simulink model "Lab1_2_Integration_RLC"  (R2024b)
settings: Solver=FixedStepAuto  StartTime=0.0  StopTime=10.0  FixedStep=1e-3  RelTol=1e-3
undefined symbols (not defined in the file or in its folder): DiscIntNeverNeededParam
libraries: simulink x1
settings Model: Creator=Ahmad  LastModifiedBy=Ahmad

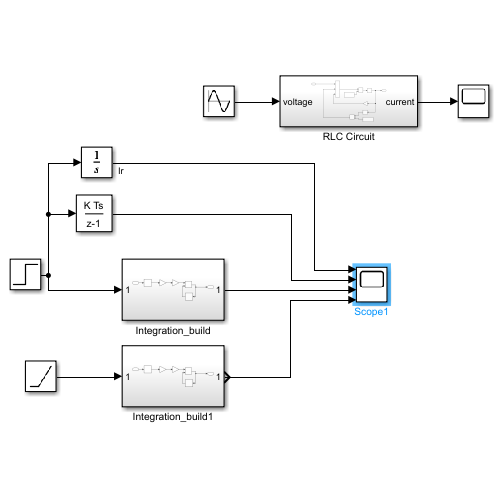
[thumbnail: Simulink's stored preview of the top-level diagram]
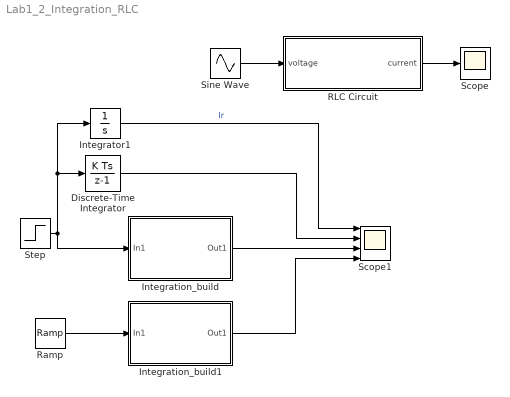
== system Lab1_2_Integration_RLC ==
  Discrete-Time Integrator : DiscreteIntegrator  SampleTime=-1  ICPrevOutput=DiscIntNeverNeededParam  ICPrevScaledInput=DiscIntNeverNeededParam
  Integration_build : Subsystem
  Integration_build1 : Subsystem
  Integrator1 : Integrator
  RLC Circuit : Subsystem
  Ramp : simulink/Sources/Ramp  slope=1  start=0  InitialOutput=0
  Scope : Scope
  Scope1 : Scope  NumInputPorts=4
  Sine Wave : Sin  SampleTime=0
  Step : Step  SampleTime=0
  wires:
  RLC Circuit/1(current) -> Scope/1
  Sine Wave/1 -> RLC Circuit/1(voltage)
  Step/1 -> Integration_build/1(In1), Discrete-Time Integrator/1, Integrator1/1
  Discrete-Time Integrator/1 -> Scope1/2
  Integrator1/1 -> Scope1/1  "Ir"
  Integration_build/1(Out1) -> Scope1/3
  Ramp/1 -> Integration_build1/1(In1)
  Integration_build1/1(Out1) -> Scope1/4

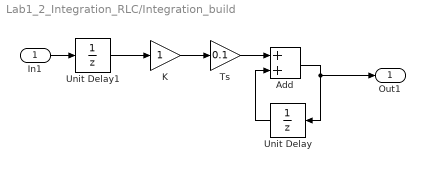
== system Lab1_2_Integration_RLC/Integration_build ==
  In1 : Inport
  Add : Sum
  K : Gain
  Ts : Gain  Gain=0.1
  Unit Delay : UnitDelay  SampleTime=-1  HasFrameUpgradeWarning=on
  Unit Delay1 : UnitDelay  SampleTime=-1  HasFrameUpgradeWarning=on
  Out1 : Outport
  wires:
  Ts/1 -> Add/1
  Unit Delay/1 -> Add/2
  In1/1 -> Unit Delay1/1
  K/1 -> Ts/1
  Add/1 -> Out1/1, Unit Delay/1
  Unit Delay1/1 -> K/1

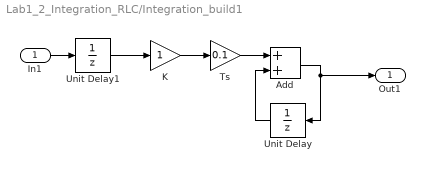
== system Lab1_2_Integration_RLC/Integration_build1 ==
  In1 : Inport
  Add : Sum
  K : Gain
  Ts : Gain  Gain=0.1
  Unit Delay : UnitDelay  SampleTime=-1  HasFrameUpgradeWarning=on
  Unit Delay1 : UnitDelay  SampleTime=-1  HasFrameUpgradeWarning=on
  Out1 : Outport
  wires:
  Ts/1 -> Add/1
  Unit Delay/1 -> Add/2
  In1/1 -> Unit Delay1/1
  K/1 -> Ts/1
  Add/1 -> Out1/1, Unit Delay/1
  Unit Delay1/1 -> K/1

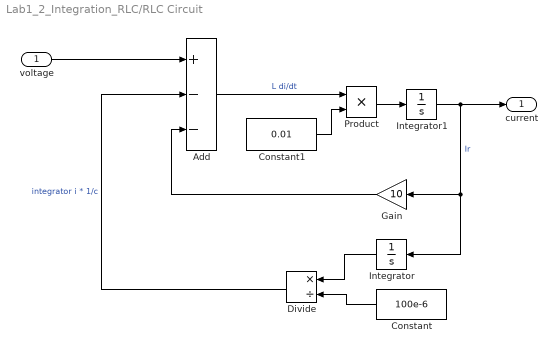
== system Lab1_2_Integration_RLC/RLC Circuit ==
  voltage : Inport
  Add : Sum  Inputs=+--
  Constant : Constant  Value=100e-6
  Constant1 : Constant  Value=0.01
  Divide : Product  Inputs=*/
  Gain : Gain  Gain=10
  Integrator : Integrator
  Integrator1 : Integrator
  Product : Product
  current : Outport
  wires:
  Product/1 -> Integrator1/1
  Add/1 -> Product/1  "L di/dt"
  Integrator1/1 -> current/1, Gain/1, Integrator/1  "Ir"
  Constant/1 -> Divide/2
  Integrator/1 -> Divide/1
  Constant1/1 -> Product/2
  Gain/1 -> Add/3
  Divide/1 -> Add/2  "integrator i * 1/c"
  voltage/1 -> Add/1
